simulink model "MPSLab1test"  (R2014b)
settings: Solver=ode45  StartTime=0.0  StopTime=30.0  RelTol=1e-3
undefined symbols (not defined in the file): magnitude
settings Model: Creator=kiril_000  LastModifiedBy=kiril_000

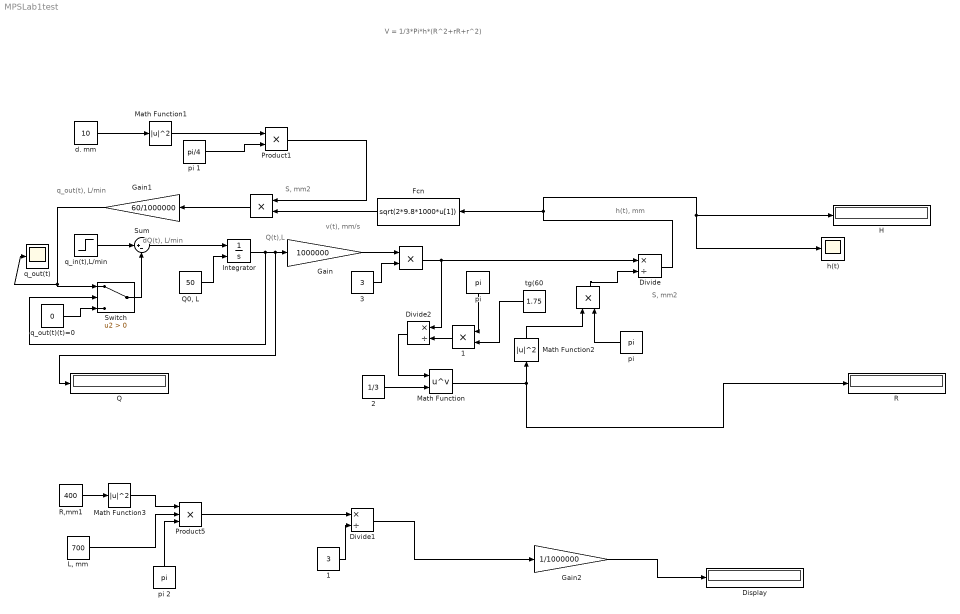
== system MPSLab1test ==
  note: h(t), mm
  note: S, mm2
  note: V = 1/3*Pi*h*(R^2+rR+r^2)
  note: v(t), mm/s
  note: q_out(t), L/min
  note: S, mm2
  note: Q(t),L
  note: dQ(t), L/min
  " " : Product
  "  " : Product
  "   " : Product
  "  1" : Product
  1 : Constant  Value=3
  2 : Constant  Value=1/3
  3 : Constant  Value=3
  Display : Display
  Divide : Product  Inputs=*/
  Divide1 : Product  Inputs=*/
  Divide2 : Product  Inputs=*/
  Fcn : Fcn  Expr=sqrt(2*9.8*1000*u[1])
  Gain : Gain  Gain=1000000
  Gain1 : Gain  Gain=60/1000000
  Gain2 : Gain  Gain=1/1000000
  H : Display
  Integrator : Integrator  InitialConditionSource=external
  "L, mm" : Constant  Value=700
  Math Function : Math  Operator=pow  SaturateOnIntegerOverflow=on
  Math Function1 : Math  Operator=magnitude^2  SaturateOnIntegerOverflow=on
  Math Function2 : Math  Operator=magnitude^2  SaturateOnIntegerOverflow=on
  Math Function3 : Math  Operator=magnitude^2  SaturateOnIntegerOverflow=on
  Product1 : Product
  Product5 : Product  Inputs=3
  Q : Display
  "Q0, L" : Constant  Value=50
  R : Display
  R,mm1 : Constant  Value=400
  Sum : Sum  Inputs=|+-
  Switch : Switch  Criteria=u2 > Threshold
  d. mm : Constant  Value=10
  h(t) : Scope
      settings: TimeRange=30  YMin=-100  YMax=600
  pi : Constant  Value=pi
  "pi " : Constant  Value=pi
  pi 1 : Constant  Value=pi/4
  pi 2 : Constant  Value=pi
  q_in(t),L/min : Step  Time=10  After=12  SampleTime=0
  q_out(t) : Scope
  q_out(t)(t)=0 : Constant  Value=0
  tg(60 : Constant  Value=1.75
  wires:
  q_in(t),L/min/1 -> Sum/1
  q_out(t)(t)=0/1 -> Switch/3
  Sum/1 -> Integrator/1
  "Q0, L"/1 -> Integrator/2
  Switch/1 -> Sum/2
  Integrator/1 -> Switch/2, Q/1, Gain/1
  Divide/1 -> Fcn/1, h(t)/1, H/1
  d. mm/1 -> Math Function1/1
  Math Function1/1 -> Product1/1
  pi 1/1 -> Product1/2
  Product1/1 -> "   "/1
  "   "/1 -> Gain1/1
  Fcn/1 -> "   "/2
  3/1 -> " "/2
  Gain/1 -> " "/1
  " "/1 -> Divide2/1, Divide/1
  "pi "/1 -> "  "/2
  "  "/1 -> Divide/2
  R,mm1/1 -> Math Function3/1
  Math Function3/1 -> Product5/1
  "L, mm"/1 -> Product5/2
  pi 2/1 -> Product5/3
  Product5/1 -> Divide1/1
  1/1 -> Divide1/2
  Divide1/1 -> Gain2/1
  Gain2/1 -> Display/1
  Math Function2/1 -> "  "/1
  Gain1/1 -> Switch/1, q_out(t)/1
  Divide2/1 -> Math Function/1
  pi/1 -> "  1"/1
  tg(60/1 -> "  1"/2
  "  1"/1 -> Divide2/2
  Math Function/1 -> R/1, Math Function2/1
  2/1 -> Math Function/2
